simulink model "seven_level"  (R2014a)
settings: Solver=ode45  StartTime=0.0  StopTime=0.1  RelTol=1e-3
values from neighbouring files (symbols this model uses):
  f5 = b    [sev_level.m]
  r5 = c    [sev_level.m]
  v5 = a    [sev_level.m]
libraries: powerlib x19
settings Model: Creator=SAMBIT  LastModifiedBy=SAMBIT

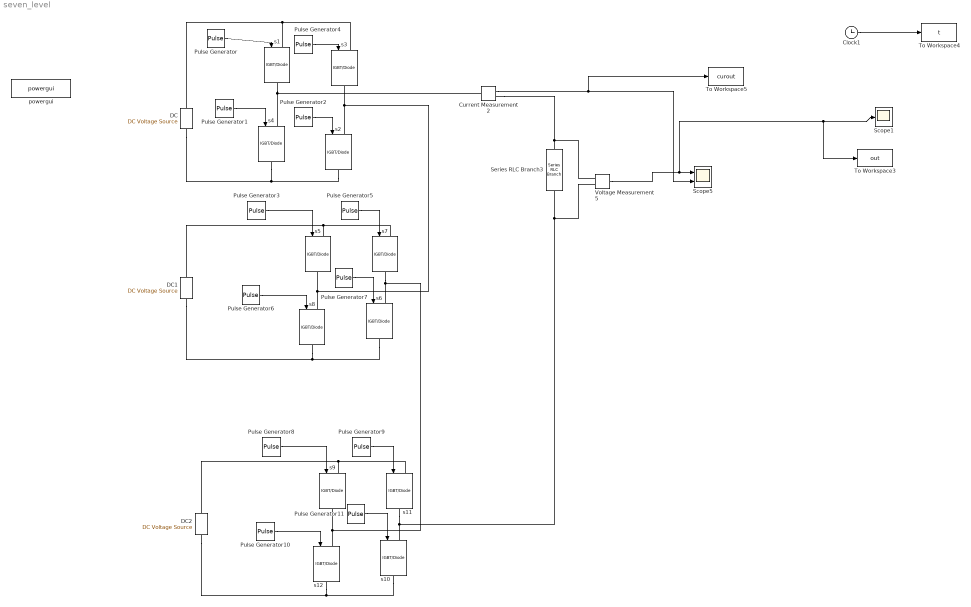
== system seven_level ==
  Clock1 : Clock
  Current Measurement2 : powerlib/Measurements/Current Measurement  PhasorSimulation=off  OutputType=Complex  PSBequivalent=0
  DC : powerlib/Electrical Sources/DC Voltage Source  Amplitude=v5  Measurements=None
  DC1 : powerlib/Electrical Sources/DC Voltage Source  Amplitude=v5  Measurements=None
  DC2 : powerlib/Electrical Sources/DC Voltage Source  Amplitude=v5  Measurements=None
  Pulse Generator{,2,7,11} (4 alike) : DiscretePulseGenerator  PulseType=Time based  Period=1/f5  PulseWidth=35.7  PhaseDelay=0.0014
  Pulse Generator{1,6,9..10} (4 alike) : DiscretePulseGenerator  PulseType=Time based  Period=1/f5  PulseWidth=35.7  PhaseDelay=0.0114
  Pulse Generator3 : DiscretePulseGenerator  PulseType=Time based  Period=1/f5  PulseWidth=21.42  PhaseDelay=0.0028
  Pulse Generator4 : DiscretePulseGenerator  PulseType=Time based  Period=1/f5  PulseWidth=7.14  PhaseDelay=0.0142
  Pulse Generator5 : DiscretePulseGenerator  PulseType=Time based  Period=1/f5  PulseWidth=21.42  PhaseDelay=0.0128
  Pulse Generator8 : DiscretePulseGenerator  PulseType=Time based  Period=1/f5  PulseWidth=7.14  PhaseDelay=0.0042
  Scope1 : Scope
  Scope5 : Scope  NumInputPorts=2
      settings: TimeRange=0.04  YMin=-1~-200  YMax=1~200  SaveName=SPBR_HL_FD  MaxDataPoints=5000000  SampleInput=on  SampleTime=5e-6
  Series RLC Branch3 : powerlib/Elements/Series RLC Branch  LConnTagsString=__new0  RConnTagsString=__new0  BranchType=R  Resistance=r5  Inductance=0  SetiL0=off  InitialCurrent=0  Capacitance=1e-6  Setx0=off  InitialVoltage=0  Measurements=None
  To Workspace3 : ToWorkspace  VariableName=out  SampleTime=-1
  To Workspace4 : ToWorkspace  VariableName=t  SampleTime=-1
  To Workspace5 : ToWorkspace  VariableName=curout  SampleTime=-1
  Voltage Measurement5 : powerlib/Measurements/Voltage Measurement  PhasorSimulation=off  OutputType=Complex  PSBequivalent=0
  powergui : powerlib/powergui  Priority=1  SimulationMode=Continuous  SolverType=Tustin  SampleTime=5e-6  frequency=60  SPID=off  DisableSnubberDevices=off  DisableRonSwitches=off  DisableVfSwitches=off  SwTol=0  Interpol=off  DisplayEquations=off  Ts=0  methode=off  frequencyindice=0  Pbase=100e6  ErrMax=1e-4  Iterations=50  UnitsV=kV  UnitsW=MW  FunctionMessages=off  echomessages=off  HookPort=off  EnableUseOfTLC=off  x0status=blocks  RestoreLinks=warning  ResistiveCurrentMeasurement=off  Frange=[0:2:500]  Ylog=off  Xlog=on  ShowGrid=off  save=off  variable=ZData  structure=SPBR_R  ZoomFFT=off  StartTime=0.0  cycles=1  DisplayStyle=1  fundamental=100  FreqAxis=off  MaxFrequency=1000  frequencyindicesteady=1  RmsSteady=1  display=off
  s{1..12} (12 alike) : powerlib/Power Electronics/IGBT//Diode  Ron=1e-3  Rs=1e5  Cs=inf  Measurements=off
  wires:
  Pulse Generator/1 -> s1/1
  Pulse Generator4/1 -> s3/1
  Pulse Generator1/1 -> s4/1
  Pulse Generator2/1 -> s2/1
  Pulse Generator6/1 -> s8/1
  Pulse Generator3/1 -> s5/1
  Pulse Generator5/1 -> s7/1
  Pulse Generator7/1 -> s6/1
  Pulse Generator10/1 -> s12/1
  Pulse Generator8/1 -> s9/1
  Pulse Generator9/1 -> s11/1
  Pulse Generator11/1 -> s10/1
  Current Measurement2/1 -> To Workspace5/1, Scope5/2
  Clock1/1 -> To Workspace4/1
  Voltage Measurement5/1 -> To Workspace3/1, Scope1/1, Scope5/1
  connections:
  s4/RConn1 -- DC/LConn1 -- s2/RConn1
  s1/LConn1 -- DC/RConn1 -- s3/LConn1
  s6/RConn1 -- DC1/LConn1 -- s8/RConn1
  s8/LConn1 -- s3/RConn1 -- s2/LConn1 -- s5/RConn1
  s5/LConn1 -- DC1/RConn1 -- s7/LConn1
  s10/RConn1 -- DC2/LConn1 -- s12/RConn1
  s12/LConn1 -- s6/LConn1 -- s7/RConn1 -- s9/RConn1
  s9/LConn1 -- DC2/RConn1 -- s11/LConn1
  s1/RConn1 -- Current Measurement2/LConn1 -- s4/LConn1
  s10/LConn1 -- s11/RConn1 -- Voltage Measurement5/LConn2 -- Series RLC Branch3/RConn1
  Current Measurement2/RConn1 -- Voltage Measurement5/LConn1 -- Series RLC Branch3/LConn1
